simulink model "time_controller_PWM"  (R2016a)
settings: Solver=VariableStepAuto  StartTime=0.0  StopTime=10  RelTol=1e-3
libraries: powerlib_meascontrol x1, powerlib x1
settings Model: Creator=villa  LastModifiedBy=villa

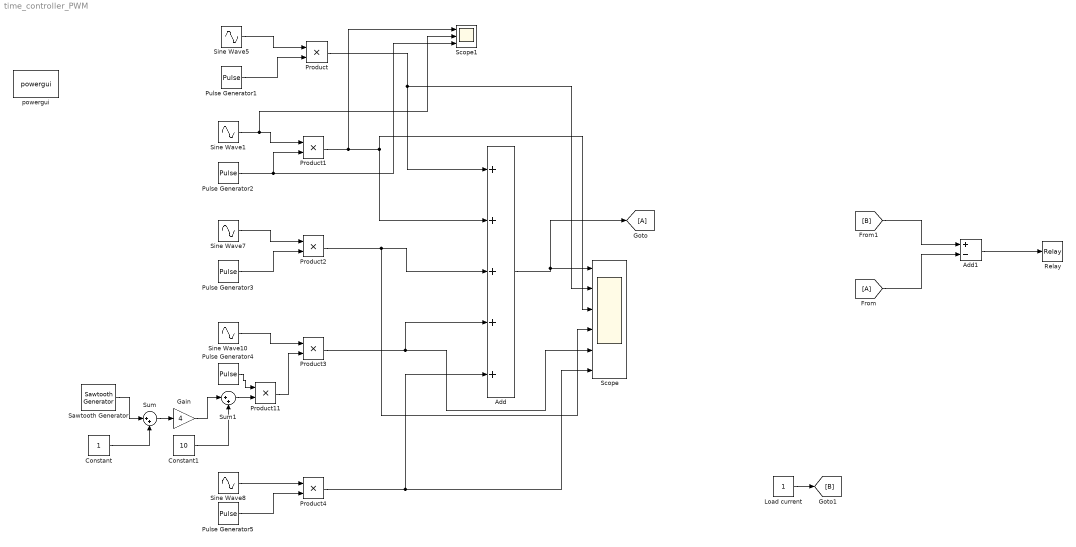
== system time_controller_PWM ==
  Add : Sum  Inputs=5
  Add1 : Sum  Inputs=+-
  Constant : Constant
  Constant1 : Constant  Value=10
  Gain : Gain  Gain=4
  Load current : Constant
  Product{,1..4,11} (6 alike) : Product
  Pulse Generator1 : DiscretePulseGenerator  PulseType=Time based  Amplitude=3  Period=6  PulseWidth=1/6*100
  Pulse Generator2 : DiscretePulseGenerator  PulseType=Time based  Amplitude=20  Period=6  PulseWidth=1/3*100  PhaseDelay=1
  Pulse Generator3 : DiscretePulseGenerator  PulseType=Time based  Amplitude=10  Period=6  PulseWidth=1/3*100  PhaseDelay=3
  Pulse Generator4 : DiscretePulseGenerator  PulseType=Time based  Period=6  PulseWidth=1/12*100  PhaseDelay=5
  Pulse Generator5 : DiscretePulseGenerator  PulseType=Time based  Amplitude=18  Period=6  PulseWidth=1/12*100  PhaseDelay=5.5
  Relay : Relay  OnSwitchValue=2  OffSwitchValue=-2
  Sawtooth Generator : powerlib_meascontrol/Pulse & Signal Generators/Sawtooth Generator  Freq=1/0.5  Phase=0  Ts=0
  Scope : Scope  NumInputPorts=6
  Scope1 : Scope  NumInputPorts=3
  Sine Wave1 : Sin  Frequency=5000/2/pi  SampleTime=0
  Sine Wave10 : Sin  Frequency=1000/2/pi  SampleTime=0
  Sine Wave5 : Sin  Frequency=500/2/pi  SampleTime=0
  Sine Wave7 : Sin  Frequency=1000/2/pi  SampleTime=0
  Sine Wave8 : Sin  Frequency=1000/2/pi  SampleTime=0
  Sum : Sum  Inputs=|++
  Sum1 : Sum  Inputs=|++
  powergui : powerlib/powergui  Priority=1  SimulationMode=Continuous  SolverType=Tustin/Backward Euler (TBE)  SampleTime=1e-7  frequency=60  SPID=off  DisableSnubberDevices=off  DisableRonSwitches=off  DisableVfSwitches=off  SwTol=0  DisplayEquations=off  Interpol=off  ExternalGateDelay=off  methode=off  Ts=10  FunctionMessages=off  echomessages=off  HookPort=off  EnableUseOfTLC=off  x0status=blocks  frequencyindice=60  Pbase=100e6  ErrMax=1e-4  Iterations=50  UnitsV=kV  UnitsW=MW  buscounter=0  RestoreLinks=warning  ResistiveCurrentMeasurement=off  Frange=[0:2:500]  Ylog=off  Xlog=on  ShowGrid=off  save=off  variable=ZData  structure=0  ZoomFFT=off  StartTime=0.0  cycles=1  DisplayStyle=1  fundamental=60  FreqAxis=off  MaxFrequency=1000  frequencyindicesteady=1  RmsSteady=1  display=off
  wires:
  Sine Wave5/1 -> Product/1
  Pulse Generator1/1 -> Product/2
  Sine Wave1/1 -> Scope1/2, Product1/1
  Pulse Generator2/1 -> Scope1/3, Product1/2
  Sine Wave7/1 -> Product2/1
  Pulse Generator3/1 -> Product2/2
  Sine Wave10/1 -> Product3/1
  Pulse Generator5/1 -> Product4/2
  Sine Wave8/1 -> Product4/1
  Pulse Generator4/1 -> Product11/1
  Sum/1 -> Gain/1
  Product11/1 -> Product3/2
  Product/1 -> Scope/2, Add/1
  Product1/1 -> Scope1/1, Add/2, Scope/3
  Product3/1 -> Scope/5, Add/4
  Product4/1 -> Scope/6, Add/5
  Add/1 -> [A], Scope/1
  Product2/1 -> Scope/4, Add/3
  Sawtooth Generator/1 -> Sum/1
  Constant/1 -> Sum/2
  Gain/1 -> Sum1/1
  Constant1/1 -> Sum1/2
  Sum1/1 -> Product11/2
  Load current/1 -> [B]
  [B] -> Add1/1
  [A] -> Add1/2
  Add1/1 -> Relay/1
